simulink model "Exp_5_3"  (R2024b)
settings: Solver=VariableStepAuto  StartTime=0.0  StopTime=10.0  RelTol=1e-3
settings Model: Creator=Rj Avro Biswas  LastModifiedBy=Rj Avro Biswas

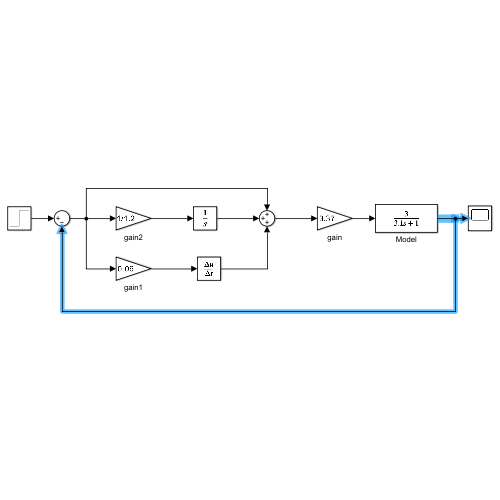
[thumbnail: Simulink's stored preview of the top-level diagram]
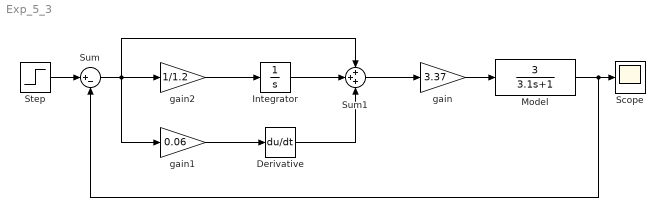
== system Exp_5_3 ==
  Derivative : Derivative
  Integrator : Integrator
  Model : TransferFcn  Numerator=3  Denominator=[3.1 1]
  Scope : Scope
  Step : Step  Time=0  After=30  SampleTime=0
  Sum : Sum  Inputs=|+-
  Sum1 : Sum  Inputs=+++
  gain : Gain  Gain=3.37
  gain1 : Gain  Gain=0.06
  gain2 : Gain  Gain=1/1.2
  wires:
  Model/1 -> Sum/2, Scope/1
  gain/1 -> Model/1
  Sum1/1 -> gain/1
  Derivative/1 -> Sum1/3
  Integrator/1 -> Sum1/2
  gain1/1 -> Derivative/1
  gain2/1 -> Integrator/1
  Sum/1 -> gain1/1, Sum1/1, gain2/1
  Step/1 -> Sum/1
